simulink model "Papersimcurrentsource1"  (R2025a)
settings: Solver=ode23tb  StartTime=0.0  StopTime=0.4  MaxStep=1e-5  RelTol=1e-3
libraries: spsRMSLib x13, spsLinearTransformerLib x3, spsParallelRLCLoadLib x3, spsCurrentMeasurementLib x2, spsThreePhaseVIMeasurementLib x2, spsVoltageMeasurementLib x2, spsACCurrentSourceLib x1, spsGroundLib x1, spsIdealSwitchLib x1, spsPower3phInstantaneousLib x1, spsThreePhasePISectionLineLib x1, spsThreePhaseSourceLib x1
settings Model: Creator=ADMIN  LastModifiedBy=ADMIN

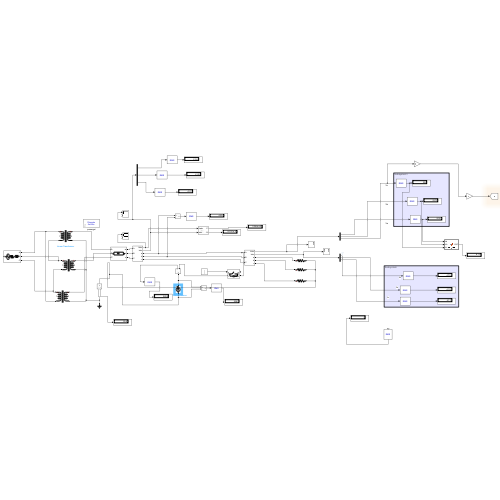
[thumbnail: Simulink's stored preview of the top-level diagram]
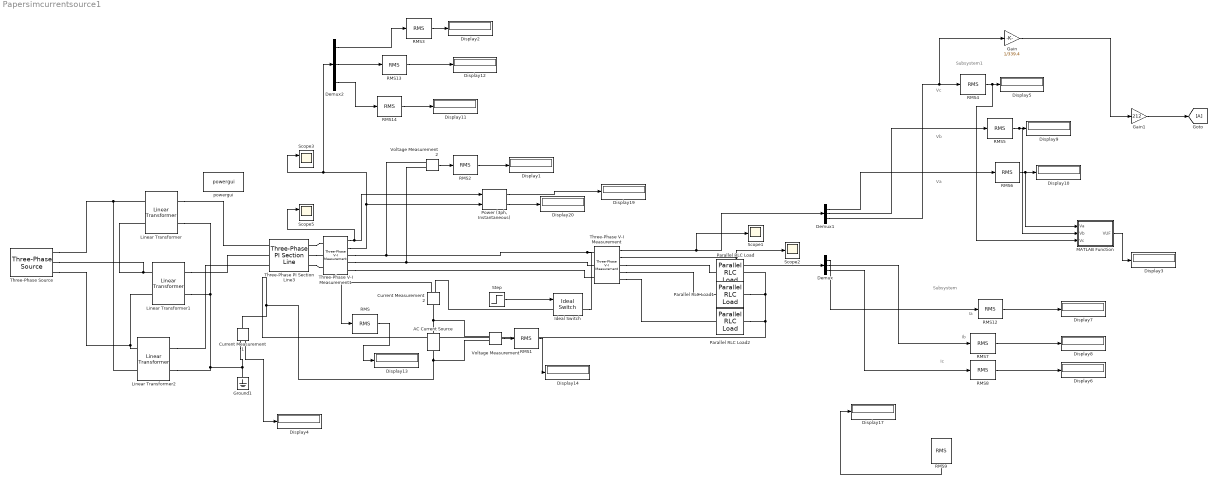
== system Papersimcurrentsource1 ==
  note: Subsystem
  note: Va
  note: Vb
  note: Vc
  note: Subsystem1
  note: Ia
  note: Ib
  note: Ic
  AC Current Source : spsACCurrentSourceLib/AC Current Source  Amplitude=354  Phase=0  Frequency=50  SampleTime=0  Measurements=None
      settings: LibrarySourceBlock=sps_lib/Sources/AC Current Source
  Current Measurement1 : spsCurrentMeasurementLib/Current Measurement  PhasorSimulation=off  OutputType=Complex  PSBequivalent=0
  Current Measurement2 : spsCurrentMeasurementLib/Current Measurement  PhasorSimulation=off  OutputType=Complex  PSBequivalent=0
  Demux : Demux  Outputs=3
  Demux1 : Demux  Outputs=3
  Demux2 : Demux  Outputs=3
  Display{1..14,17,19..20} (17 alike) : Display
  Gain : Gain  Gain=1/339.4
  Gain1 : Gain  Gain=212
  Goto : Goto
  Ground1 : spsGroundLib/Ground  LConnTagsString=a
  Ideal Switch : spsIdealSwitchLib/Ideal Switch  Ron=0.001  Lon=0  IC=0  Rs=1e5  Cs=inf  Measurements=on
  Linear Transformer : spsLinearTransformerLib/Linear Transformer  UNITS=pu  NominalPower="[66.67e3  50 ]"  winding1="[ 11000  0.01  0.08 ]"  winding2="[ 239.6  0.01  0.08 ]"  ThreeWindings=off  winding3=[ 315e3 0.002 0.08 ]  RmLm=[ 500 500 ]  Measurements=None  DataType=off
  Linear Transformer1 : spsLinearTransformerLib/Linear Transformer  UNITS=pu  NominalPower=[ 66.67e3 50 ]  winding1="[11000  0.01  0.08 ]"  winding2="[ 239.6  0.01  0.08 ]"  ThreeWindings=off  winding3=[ 315e3 0.002 0.08 ]  RmLm=[ 500 500 ]  Measurements=None  DataType=off
  Linear Transformer2 : spsLinearTransformerLib/Linear Transformer  UNITS=pu  NominalPower=[ 66.67e3 50 ]  winding1="[11000  0.01  0.08 ]"  winding2="[ 239.6  0.01  0.08 ]"  ThreeWindings=off  winding3=[ 315e3 0.002 0.08 ]  RmLm=[ 500 500 ]  Measurements=None  DataType=off
  MATLAB Function : MATLAB Function  TreatAsAtomicUnit=on
  Parallel RLC Load : spsParallelRLCLoadLib/Parallel RLC Load  LConnTagsString=a  RConnTagsString=__new0  NominalVoltage=239.6  NominalFrequency=50  ActivePower=10e3  InductivePower=0  CapacitivePower=0  Setx0=off  InitialVoltage=0  SetiL0=off  InitialCurrent=0  Measurements=None  LoadType=constant Z
      settings: AttributesFormatString=\n  LibrarySourceBlock=sps_lib/Passives/Parallel RLC Load
  Parallel RLC Load1 : spsParallelRLCLoadLib/Parallel RLC Load  LConnTagsString=a  RConnTagsString=__new0  NominalVoltage=239.6  NominalFrequency=50  ActivePower=10e3  InductivePower=0  CapacitivePower=0  Setx0=off  InitialVoltage=0  SetiL0=off  InitialCurrent=0  Measurements=None  LoadType=constant Z
      settings: AttributesFormatString=\n  LibrarySourceBlock=sps_lib/Passives/Parallel RLC Load
  Parallel RLC Load2 : spsParallelRLCLoadLib/Parallel RLC Load  LConnTagsString=a  RConnTagsString=__new0  NominalVoltage=239.6  NominalFrequency=50  ActivePower=10e3  InductivePower=0  CapacitivePower=0  Setx0=off  InitialVoltage=0  SetiL0=off  InitialCurrent=0  Measurements=None  LoadType=constant Z
      settings: AttributesFormatString=\n  LibrarySourceBlock=sps_lib/Passives/Parallel RLC Load
  "Power (3ph, Instantaneous)" : spsPower3phInstantaneousLib/Power (3ph, Instantaneous)
  RMS : spsRMSLib/RMS  TrueRMS=on  Freq=60  RMSInit=120  Ts=0
  RMS1 : spsRMSLib/RMS  TrueRMS=on  Freq=60  RMSInit=120  Ts=0
  RMS{2..9,12..14} (11 alike) : spsRMSLib/RMS  TrueRMS=on  Freq=50  RMSInit=120  Ts=0
  Scope1 : Scope
      settings: ActiveDisplayYMinimum=203.11451236491536  ActiveDisplayYMaximum=759.75565775064547
  Scope2 : Scope
      settings: ActiveDisplayYMinimum=166.80982141705707  ActiveDisplayYMaximum=205.76032421549655  DataLoggingVariableName=ScopeData2
  Scope3 : Scope  NumInputPorts=2
      settings: ActiveDisplayYMinimum=512.348102583599  ActiveDisplayYMaximum=514.20096322187453
  Scope5 : Scope  NumInputPorts=2
      settings: ActiveDisplayYMinimum=-117.5320725063296  ActiveDisplayYMaximum=475.83225268630645  DataLoggingVariableName=ScopeData4
  Step : Step  Time=0.2  SampleTime=5e-6
  Three-Phase PI Section Line3 : spsThreePhasePISectionLineLib/Three-Phase PI Section Line  LConnTagsString=a|b|c  RConnTagsString=A|B|C  Length=1.2  Frequency=50  Resistances=[0.01377 0.04131 ]  Inductances=[31.83e-6 95.49e-6]  Capacitances=[250e-9 80e-9]
  Three-Phase V-I Measurement : spsThreePhaseVIMeasurementLib/Three-Phase V-I Measurement  VoltageMeasurement=phase-to-ground  SetLabelV=off  LabelV=Vabc  Vpu=off  VpuLL=off  CurrentMeasurement=yes  SetLabelI=off  LabelI=Iabc  Ipu=off  Pbase=100e6  Vbase=500e3  OutputType=Complex  PhasorSimulation=off  PSBequivalent=0
  Three-Phase V-I Measurement1 : spsThreePhaseVIMeasurementLib/Three-Phase V-I Measurement  VoltageMeasurement=phase-to-ground  SetLabelV=off  LabelV=Vabc  Vpu=off  VpuLL=off  CurrentMeasurement=yes  SetLabelI=off  LabelI=Iabc  Ipu=off  Pbase=100e6  Vbase=500e3  OutputType=Complex  PhasorSimulation=off  PSBequivalent=0
  Three-Phase Source : spsThreePhaseSourceLib/Three-Phase Source  InternalConnection=Yn  VoltagePhases=off  Voltage=11000  PhaseAngle=0  Voltage_phases=[25e3 25e3 25e3]/sqrt(3)  PhaseAngles_phases=[0 -120 +120]  Frequency=50  NonIdealSource=on  SpecifyImpedance=on  Resistance=0.01  Inductance=0.1  ShortCircuitLevel=10e6  BaseVoltage=11e3  XRratio=7  BusType=swing  Pref=10e3  Qref=0  Prefabc=[10e3, 10e3, 10e3]  Qrefabc=[0, 0, 0]  Qmin=-inf  Qmax=inf
  Voltage Measurement : spsVoltageMeasurementLib/Voltage Measurement  PhasorSimulation=off  OutputType=Complex  PSBequivalent=0
  Voltage Measurement2 : spsVoltageMeasurementLib/Voltage Measurement  PhasorSimulation=off  OutputType=Complex  PSBequivalent=0
  powergui : sps_lib/powergui  Priority=1  SimulationMode=Discrete  SampleTime=5e-6  frequency=50  Iterations=50  frequencyindice=50  Pbase=100e6  ErrMax=1e-4  UnitsV=kV  UnitsW=MW  buscounter=0  FunctionMessages=off  echomessages=off  EnableUseOfTLC=off  CurrentSourceSwitches=off  DisableSnubberDevices=off  DisableRonSwitches=off  DisableVfSwitches=off  DisplayEquations=off  AutomaticDiscreteSolvers=off  SolverType=Tustin/Backward Euler (TBE)  Interpol=off  ExternalGateDelay=off  methode=off  Ts=100  x0status=blocks  SPID=on  SwTol=0  HookPort=off  NonlinearTolerance=1e-4  nMaxIteration=100  ContinueOnMaxIteration=off  RestoreLinks=warning  ResistiveCurrentMeasurement=off  Frange=[0:2:500]  Ylog=off  Xlog=on  ShowGrid=off  save=off  variable=ZData  structure=0  ZoomFFT=off  StartTime=0.0  cycles=1  DisplayStyle=1  fundamental=60  FreqAxis=off  MaxFrequency=1000  frequencyindicesteady=1  RmsSteady=1  display=off
  wires:
  Voltage Measurement2/1 -> RMS2/1
  RMS2/1 -> Display1/1
  Three-Phase V-I Measurement/1 -> Demux1/1, Scope1/1
  Three-Phase V-I Measurement/2 -> Scope2/1, Demux/1
  Current Measurement1/1 -> Display4/1
  Demux1/2 -> RMS5/1
  Demux1/3 -> Gain/1, RMS4/1
  Demux1/1 -> RMS6/1
  RMS4/1 -> MATLAB Function/3(Vc), Display5/1
  RMS6/1 -> MATLAB Function/1(Va), Display10/1
  RMS5/1 -> MATLAB Function/2(Vb), Display9/1
  MATLAB Function/1(VUF) -> Display3/1
  Demux/3 -> RMS8/1
  Demux/1 -> RMS12/1
  Demux2/2 -> RMS13/1
  Demux2/3 -> RMS14/1
  Three-Phase V-I Measurement1/2 -> "Power (3ph, Instantaneous)"/2, Scope3/1, Demux2/1
  Three-Phase V-I Measurement1/1 -> Scope5/1, "Power (3ph, Instantaneous)"/1
  Demux/2 -> RMS7/1
  RMS7/1 -> Display8/1
  RMS8/1 -> Display6/1
  RMS14/1 -> Display11/1
  RMS13/1 -> Display12/1
  Demux2/1 -> RMS3/1
  RMS3/1 -> Display2/1
  RMS9/1 -> Display17/1
  RMS12/1 -> Display7/1
  Gain/1 -> Gain1/1
  Gain1/1 -> Goto/1
  "Power (3ph, Instantaneous)"/2 -> Display20/1
  "Power (3ph, Instantaneous)"/1 -> Display19/1
  Current Measurement2/1 -> RMS/1
  RMS/1 -> Display13/1
  Voltage Measurement/1 -> RMS1/1
  RMS1/1 -> Display14/1
  Step/1 -> Ideal Switch/1
  connections:
  Current Measurement1/LConn1 -- Parallel RLC Load1/RConn1 -- Parallel RLC Load/RConn1 -- Parallel RLC Load2/RConn1 -- Voltage Measurement/LConn2 -- AC Current Source/LConn1
  Linear Transformer/RConn2 -- Linear Transformer1/RConn2 -- Linear Transformer2/RConn2 -- Ground1/LConn1 -- Current Measurement1/RConn1
  Three-Phase V-I Measurement1/RConn3 -- Three-Phase V-I Measurement/LConn3
  Voltage Measurement2/LConn2 -- Three-Phase V-I Measurement/LConn2 -- Three-Phase V-I Measurement1/RConn2
  Three-Phase PI Section Line3/RConn3 -- Three-Phase V-I Measurement1/LConn3
  Three-Phase PI Section Line3/RConn2 -- Three-Phase V-I Measurement1/LConn2
  Three-Phase PI Section Line3/RConn1 -- Three-Phase V-I Measurement1/LConn1
  Three-Phase V-I Measurement/RConn1 -- Parallel RLC Load/LConn1
  AC Current Source/RConn1 -- Current Measurement2/LConn1 -- Voltage Measurement/LConn1
  Three-Phase V-I Measurement/RConn2 -- Parallel RLC Load1/LConn1
  Three-Phase V-I Measurement/RConn3 -- Parallel RLC Load2/LConn1
  Ideal Switch/LConn1 -- Current Measurement2/RConn1
  Three-Phase V-I Measurement1/RConn1 -- Voltage Measurement2/LConn1 -- Ideal Switch/RConn1 -- Three-Phase V-I Measurement/LConn1
  Three-Phase Source/RConn1 -- Linear Transformer2/LConn2 -- Linear Transformer/LConn1
  Linear Transformer/LConn2 -- Three-Phase Source/RConn2 -- Linear Transformer1/LConn1
  Linear Transformer1/LConn2 -- Three-Phase Source/RConn3 -- Linear Transformer2/LConn1
  Linear Transformer/RConn1 -- Three-Phase PI Section Line3/LConn1
  Linear Transformer1/RConn1 -- Three-Phase PI Section Line3/LConn2
  Linear Transformer2/RConn1 -- Three-Phase PI Section Line3/LConn3

== matlab function Papersimcurrentsource1/MATLAB Function ==
  data: Va input; VUF output; Vb input; Vc input
function VUF = calc_VUF(Va, Vb, Vc)

Vavg = (Va + Vb + Vc)/3;

devA = abs(Va - Vavg);
devB = abs(Vb - Vavg);
devC = abs(Vc - Vavg);

max_dev = max([devA, devB, devC]);

VUF = (max_dev / Vavg) * 100;

end
